simulink model "CRCL"  (R2020b)
settings: Solver=FixedStepDiscrete  StartTime=0.0  StopTime=inf  FixedStep=0.01  RelTol=1e-3  EnableMultiTasking=on
values from neighbouring files (symbols this model uses):
  calibrationDelayTime_s = 2.0    [CRCL_Dictionary.sldd]
  collisionAngleThreshold_deg = 40.0    [CRCL_Dictionary.sldd]
  collisionVarianceThreshold_g2 = 8.0    [CRCL_Dictionary.sldd]
  cpMaxAbortTime_s = 30.0    [CRCL_Dictionary.sldd]
  cpMaxTipOverAngle_deg = 35.0    [CRCL_Dictionary.sldd]
  cpMinEstDistance_m = 50.0    [CRCL_Dictionary.sldd]
  cpMinEstDistanceGnssBased_m = 200.0    [CRCL_Dictionary.sldd]
  cpMinRiddenTime_s = 15.0    [CRCL_Dictionary.sldd]
  cpMinSpeedRiding_kmh = 10.0    [CRCL_Dictionary.sldd]
  cpNumCrankRevolutionThreshold = 5.0    [CRCL_Dictionary.sldd]
  cpSpeedCond2PositiveSpeedChangeTime_s = 5.0    [CRCL_Dictionary.sldd]
  cpSpeedDerivativeThreshold_kmhs = 0.005    [CRCL_Dictionary.sldd]
  cpTimeOutSpeedCond2_s = 15.0    [CRCL_Dictionary.sldd]
  groundHitEnergyThresholdStanding_g2s2 = 0.02    [CRCL_Dictionary.sldd]
  groundHitTipOverAngleThreshold_deg = 40.0    [CRCL_Dictionary.sldd]
  longAccCompForEulerEstFlag = 0.0    [CRCL_Dictionary.sldd]
  minEnergyStrongHit_g2s2 = 0.1    [CRCL_Dictionary.sldd]
  noMotionAccVarianceThresholdSD_g2 = 0.001    [CRCL_Dictionary.sldd]
  ride1minSpeedSlow_kmh = 4.0    [CRCL_Dictionary.sldd]
  ride2minSpeed_kmh = 8.0    [CRCL_Dictionary.sldd]
  rroMaxSpeed_kmh = 5.0    [CRCL_Dictionary.sldd]
  rroMinGyrX_degs = 20.0    [CRCL_Dictionary.sldd]
  rroMonotonyThreshold_degs = -1.0    [CRCL_Dictionary.sldd]
  rroRollIntegrationAngleThreshold_degs = 20.0    [CRCL_Dictionary.sldd]
  rroUniContinuityThreshold_degs = 15.0    [CRCL_Dictionary.sldd]
  scaleFactorVarianceStrongHit = 2.0    [CRCL_Dictionary.sldd]
  sdoMaxAccVarFreeFall_g2 = 0.06    [CRCL_Dictionary.sldd]
  sdoMaxTipOverAngle_deg = 20.0    [CRCL_Dictionary.sldd]
  sdoMinAccVar_g2 = 8.0    [CRCL_Dictionary.sldd]
  sdoMinGyrXYNorm_degs = 720.0    [CRCL_Dictionary.sldd]
  sdoMinGyrXYNormFreeFall_degs = 100.0    [CRCL_Dictionary.sldd]
  sdoMinOrientationChange_deg = 120.0    [CRCL_Dictionary.sldd]
  sdoScaleFactorOrientationChange = 3.0    [CRCL_Dictionary.sldd]
  stepTime_s = 0.01    [CRCL_Dictionary.sldd]
  strongHitSafetyFactor = 2.5    [CRCL_Dictionary.sldd]
  tipOverAccZFiltTreshold_g = 0.7    [CRCL_Dictionary.sldd]
  tipOverAngleThreshold_deg = 50.0    [CRCL_Dictionary.sldd]
  tipOverMinAccZFiltNoseOver_g = 0.3    [CRCL_Dictionary.sldd]
  tipOverRollPitchRelationNoseOver = 1.5    [CRCL_Dictionary.sldd]
undefined symbols (not defined in the file or in its folder): magnitude
libraries: simulink x17
(part 1 of 8)
settings Model: DataDictionary=CRCL_Dictionary.sldd  EnableAccessToBaseWorkspace=off  DataTypeOverride=Off  DataTypeOverrideAppliesTo=Floating-point  MinMaxOverflowLogging=ForceOff  Creator=stj1si  LastModifiedBy=HNA3SI
settings DataIOCC: SaveFormat=Array  SaveOutput=off  SaveTime=off  ReturnWorkspaceOutputs=off
settings OptimizationCC: DefaultParameterBehavior=Inlined  DefaultUnderspecifiedDataType=single  InlineInvariantSignals=on  EnhancedBackFolding=on  CachingGlobalReferences=on  ExpressionDepthLimit=2147483647  NoFixptDivByZeroProtection=on  EfficientFloat2IntCast=on  LifeSpan=1  SimCompilerOptimization=on  EfficientTunableParamExpr=on
settings DebuggingCC: SolverPrmCheckMsg=warning  ParameterPrecisionLossMsg=none  AllowSymbolicDim=off  StateNameClashWarn=warning  SFUnexpectedBacktrackingDiag=warning  SFNoUnconditionalDefaultTransitionDiag=warning  SFExecutionAtInitializationDiag=none  UnderSpecifiedDimensionMsg=warning  ArithmeticOperatorsInVariantConditions=warning
settings HardwareCC: ProdBitPerPointer=32  ProdBitPerSizeT=32  ProdBitPerPtrDiffT=32  ProdLargestAtomicInteger=Long  ProdLargestAtomicFloat=Double  ProdEndianess=BigEndian  ProdWordSize=32  ProdHWDeviceType=Freescale->32-bit PowerPC
settings ModelReferenceCC: ModelReferenceNumInstancesAllowed=Single  PropagateSignalLabelsOutOfModel=off
settings SFSimCC: SimUseLocalCustomCode=off  MATLABDynamicMemAlloc=off  CustomCodeUndefinedFunction=UseInterfaceOnly
settings RTWCC: Description=Embedded Coder  SystemTargetFile=ert.tlc  GenCodeOnly=on  TemplateMakefile=ert_default_tmf  GenerateReport=on  RTWUseLocalCustomCode=off  IncludeHyperlinkInReport=on  LaunchReport=on  GenerateTraceInfo=on  GenerateTraceReport=on  GenerateTraceReportSl=on  GenerateTraceReportSf=on  GenerateTraceReportEml=on
settings CodeAppCC: IgnoreCustomStorageClasses=off  CustomSymbolStrType=$N$R$M  CustomSymbolStrBlkIO=SMON_rtb_$N$M  StateflowObjectComments=on  InternalIdentifier=Classic
settings ERTTargetCC: TargetLangStandard=C99 (ISO)  MultiwordLength=2048  GenerateSampleERTMain=on  IncludeMdlTerminateFcn=off  CombineSignalStateStructs=on  SuppressErrorStatus=on  SupportNonFinite=off  SupportComplex=off  CastingMode=Standards  InlinedParameterPlacement=NonHierarchical  ERTSrcFileBannerTemplate=ert_code_template_ebike.cgt  ERTCustomFileTemplate=example_file_process.tlc  ERTFilePackagingFormat=Compact  PreserveExternInFcnDecls=off  SuppressUnreachableDefaultCases=off  EnableSignedLeftShifts=off  EnableSignedRightShifts=off  IndentStyle=Allman  EnableUserReplacementTypes=on
settings ConfigComp: CovEnable=on  CovScope=ReferencedModels  CovIncludeTopModel=off  CovMetricSettings=dw  CovHTMLOptions=-sRT=1 -sVT=0 -aTS=1 -bRG=1 -bTC=1 -hTR=0 -nFC=0 -nFD=1 -scm=1 -bcm=1 -xEv=0 -xEM=0  CovSaveCumulativeToWorkspaceVar=on  CovSaveSingleToWorkspaceVar=on  CovModelRefEnable=all  CovSFcnEnable=off

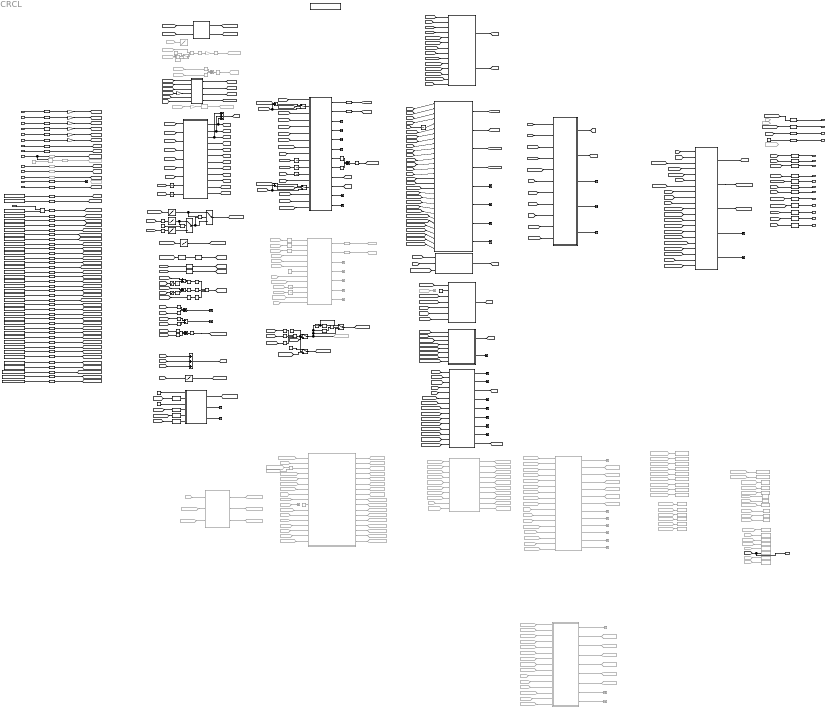
== system CRCL ==
  note: // hub setup (2==smarphoneHub, 1==bio bike cobi pro, 0==eBike cobi pro)
  note: remove speed jumps to 0km/h (FP Tobi 2021_03_30)
  note: set initially to 0.01s
  note: not used atm!
  note: RideDetection
  note: TipOverDetection
  note: HitAndStandDetection
  note: CrashFusion
  note: RiderlessRollOver
  note: SmartphoneDropOutDetection
  note: pass only current speed value, if hub Connection is available ( in eBike cobi use case)
  note: set initially to 2s
  note: set initially to 0 -> off
  note: set initially to 50°
  note: set initially to 0.3g
  note: set initially to 0.7g
  note: set initially to 1.5
  note: Cobi: set initially to 0.02
      | DU: set initially to 0.015 -> update!
  note: set initially to 40°
  note: set initially to 8g²
  note: Cobi: set initially to 2.5
      | DU: set initially to 3
  note: set initially to 2
  note: set initially to 0.1
  note: set initially to 40°
  note: set initially to 0.001 g²
  note: set initially to 4km/h
  note: set initially to 8km/h
  note: set initially to 20 °/s
  note: set initially to 15 °/s
  note: set initially to 5km/h
  note: set initially to -1°/s
  note: set initially to 20 °/s
  note: set initially to 20°
  note: set initially to 8g²
  note: set initially to 720°/s
  note: set initially to 120°
  note: set initially to 3
  note: set initially to 0.06g²
  note: set initially to 100°/s
  note: set initially to 5s
  note: set initially to 15s
  note: set initially to 15s
  note: set initially to 30s
  note: set initially to 5
  note: set initially to 200m
  note: set initially to 3 kmh
  note: set initially to 0.005 km/(h*s)
  note: set initially to 35°
  note: AVOID DIVISION BY ZERO!
  note: AVOID DIVISION BY ZERO!
  note: REMOVED DIVISION BY ZERO!
  note: Division by 0 possible!!!
  note: Division by 0 possible!!!
  note: AVOID DIVISION BY ZERO!
  note: not used atm!
  note: pass only current speed value, if hub Connection is avaiable ( in eBike cobi use case)
  note: set initially to 50m
  note: SystemConfig == 1 -> drive unit, SystemConfig == 2 -> all other
  acc_x [mg] : Inport  PortDimensions=1
  acc_y [mg] : Inport  Port=2  PortDimensions=1
  acc_z [mg] : Inport  Port=3  PortDimensions=1
  gyr_x [mdeg/s] : Inport  Port=4  PortDimensions=1
  gyr_y [mdeg/s] : Inport  Port=5  PortDimensions=1
  gyr_z [mdeg/s] : Inport  Port=6  PortDimensions=1
  DU_cadence [rpm] : Inport  Port=7  PortDimensions=1
  DU_Speed [kmh] : Inport  Port=8  PortDimensions=1
  SecondCalibDone : Inport  Port=9  PortDimensions=1
  SystemConfig [1/2] : Inport  Port=10  PortDimensions=1
  CobiHubConnection [0/1] : Inport  Port=11  PortDimensions=1
  cobiSetup [0/1/2] : Inport  Port=12  PortDimensions=1
  accDuX [mg] : Inport  Port=13  PortDimensions=1
  accDuZ [mg] : Inport  Port=14  PortDimensions=1
  speedCompFlag [0/1] : Inport  Port=15  PortDimensions=1
  1-D Lookup Table : Lookup_n-D  Commented=on  NumberOfTableDimensions=1  BreakpointsForDimension1=[1 2 3 4 5 6 7]  Table=[2 15 3 15 3 15 2]  ExtrapMethod=Clip  InternalRulePriority=Speed  RndMeth=Simplest  InputSameDT=on
  1-D Lookup Table1 : Lookup_n-D  NumberOfTableDimensions=1  BreakpointsForDimension1=[0 9000 10000 15000 30000 100000]  Table=[1 1 0.75 0.5 0.3 0.3]  InternalRulePriority=Speed  RndMeth=Simplest  InputSameDT=on
  1-D Lookup Table2 : Lookup_n-D  NumberOfTableDimensions=1  BreakpointsForDimension1=[0 20 35 45 50 90]  Table=[0.015 0.015 0.04 0.04 0.5 0.5]  InternalRulePriority=Speed  RndMeth=Simplest  InputSameDT=on
  1-D Lookup Table3 : Lookup_n-D  NumberOfTableDimensions=1  BreakpointsForDimension1=[0:100]  Table=-1./exp(0.09*[0:100]+3.5) + 0.045  InternalRulePriority=Speed  RndMeth=Simplest  InputSameDT=on
  1-D Lookup Table4 : Lookup_n-D  NumberOfTableDimensions=1  BreakpointsForDimension1=[0 20 45 60 180]  Table=[1 1 0.03 0.01 0.01]  InternalRulePriority=Speed  RndMeth=Simplest  InputSameDT=on
  1-D Lookup Table5 : Lookup_n-D  NumberOfTableDimensions=1  BreakpointsForDimension1=[0 15 25 90]  Table=[0.015 0.015 0.04 0.04]  InternalRulePriority=Speed  RndMeth=Simplest  InputSameDT=on
  Abs{,1..3,5} (5 alike) : Abs
  Abs4 : Abs  Commented=on
  Add : Sum  Inputs=+-
  Add1 : Sum  Inputs=+++
  Add10 : Sum  Inputs=-+
  Add2 : Sum  Commented=on
  Add{3..5,9} (4 alike) : Sum
  Add6 : Sum  Inputs=-+
  Add7 : Sum  Inputs=+++
  Add8 : Sum  Inputs=+-
  Atan : Trigonometry  Commented=on  Operator=atan
  BikeCrashFusionProduct : Stateflow chart  TreatAsAtomicUnit=on
  CP_crashPlausiblizer : Stateflow chart  TreatAsAtomicUnit=on
  Chart : Stateflow chart  TreatAsAtomicUnit=on
  Chart1 : Stateflow chart  TreatAsAtomicUnit=on
  Chart2 : Stateflow chart  Commented=on  TreatAsAtomicUnit=on
  Chart3 : Stateflow chart  Commented=on  TreatAsAtomicUnit=on
  Compare To Constant : simulink/Logic and Bit Operations/Compare To Constant  relop=>=  const=3  OutDataTypeStr=boolean
  Compare To Constant1 : simulink/Logic and Bit Operations/Compare To Constant  relop=>=  const=3  OutDataTypeStr=boolean
  Compare To Constant2 : simulink/Logic and Bit Operations/Compare To Constant  relop=>=  const=3  OutDataTypeStr=boolean
  Compare To Constant3 : simulink/Logic and Bit Operations/Compare To Constant  relop=<=  const=0.1  OutDataTypeStr=boolean
  Compare To Constant4 : simulink/Logic and Bit Operations/Compare To Constant  relop=>=  const=10  OutDataTypeStr=boolean
  Compare To Constant6 : simulink/Logic and Bit Operations/Compare To Constant  relop===  const=0  OutDataTypeStr=boolean
  Compare To Constant7 : simulink/Logic and Bit Operations/Compare To Constant  relop===  const=2  OutDataTypeStr=boolean
  Compare To Constant8 : simulink/Logic and Bit Operations/Compare To Constant  relop=~=  const=1  OutDataTypeStr=boolean
  Compare To Constant9 : simulink/Logic and Bit Operations/Compare To Constant  Commented=on  relop===  const=0  OutDataTypeStr=boolean
  Constant : Constant  Commented=on  Value=0.02  OutDataTypeStr=single
  Constant{1,7,9,11} (4 alike) : Constant  Value=0
  Constant10 : Constant  Value=tipOverAccZFiltTreshold_g
  Constant12 : Constant  Value=tipOverMinAccZFiltNoseOver_g
  Constant13 : Constant  Value=tipOverRollPitchRelationNoseOver
  Constant14 : Constant  Value=groundHitEnergyThresholdStanding_g2s2
  Constant15 : Constant  Value=minEnergyStrongHit_g2s2
  Constant16 : Constant  Value=collisionAngleThreshold_deg
  Constant17 : Constant  Value=noMotionAccVarianceThresholdSD_g2
  Constant18 : Constant  Value=ride1minSpeedSlow_kmh
  Constant19 : Constant  Value=groundHitTipOverAngleThreshold_deg
  Constant2 : Constant  Value=stepTime_s
  Constant20 : Constant  Value=collisionVarianceThreshold_g2
  Constant21 : Constant  Value=strongHitSafetyFactor
  Constant22 : Constant  Value=scaleFactorVarianceStrongHit
  Constant23 : Constant  Value=rroMonotonyThreshold_degs
  Constant24 : Constant  Value=rroRollIntegrationAngleThreshold_degs
  Constant25 : Constant  Value=sdoMaxTipOverAngle_deg
  Constant26 : Constant  Value=sdoMinAccVar_g2
  Constant27 : Constant  Value=sdoMinGyrXYNormFreeFall_degs
  Constant28 : Constant  Value=cpMaxAbortTime_s
  Constant29 : Constant  Value=cpMinSpeedRiding_kmh
  Constant3 : Constant  Value=calibrationDelayTime_s
  Constant30 : Constant  Value=cpNumCrankRevolutionThreshold
  Constant31 : Constant  Value=sdoMinGyrXYNorm_degs
  Constant32 : Constant  Value=ride2minSpeed_kmh
  Constant33 : Constant  Value=sdoMinOrientationChange_deg
  Constant34 : Constant  Value=sdoScaleFactorOrientationChange
  Constant35 : Constant  Value=sdoMaxAccVarFreeFall_g2
  Constant36 : Constant  Value=rroMinGyrX_degs
  Constant37 : Constant  Value=rroUniContinuityThreshold_degs
  Constant38 : Constant  Value=rroMaxSpeed_kmh
  Constant39 : Constant  Value=cpTimeOutSpeedCond2_s
  Constant4 : Constant  Commented=on
  Constant40 : Constant  Value=cpSpeedCond2PositiveSpeedChangeTime_s
  Constant41 : Constant  Value=cpSpeedDerivativeThreshold_kmhs
  Constant42 : Constant  Value=cpMaxTipOverAngle_deg
  Constant43 : Constant  Value=cpMinEstDistance_m
  Constant44 : Constant  Value=cpMinRiddenTime_s
  Constant45 : Constant  Commented=on  Value=0
  Constant46 : Constant  Value=10
  Constant47 : Constant  Value=0.1
  Constant48 : Constant  Commented=on  Value=0.001  OutDataTypeStr=single
  Constant49 : Constant  Value=0  OutDataTypeStr=single
  Constant5 : Constant  Value=longAccCompForEulerEstFlag
  Constant6 : Constant  Value=tipOverAngleThreshold_deg
  Constant8 : Constant  Value=cpMinEstDistanceGnssBased_m
  Data Type Conversion{,19,21,23..24,27..33} (12 alike) : DataTypeConversion  RndMeth=Zero
  Data Type Conversion{1..4,6..9,12..14,18,20,22,34..36,40,42..74,76..77} (53 alike) : DataTypeConversion  OutDataTypeStr=single
  Data Type Conversion10 : DataTypeConversion  RndMeth=Simplest
  Data Type Conversion11 : DataTypeConversion  OutDataTypeStr=int16
  Data Type Conversion15 : DataTypeConversion  OutDataTypeStr=Enum: CrashClass  RndMeth=Simplest
  Data Type Conversion16 : DataTypeConversion  RndMeth=Simplest
  Data Type Conversion17 : DataTypeConversion  RndMeth=Simplest
  Data Type Conversion25 : DataTypeConversion  Commented=on  OutDataTypeStr=single
  Data Type Conversion26 : DataTypeConversion  Commented=on  OutDataTypeStr=single
  Data Type Conversion{37..39,41} (4 alike) : DataTypeConversion  Commented=through  OutDataTypeStr=single
  Data Type Conversion5 : DataTypeConversion  Commented=on  OutDataTypeStr=single
  Data Type Conversion75 : DataTypeConversion  OutDataTypeStr=int16
  Discrete Derivative : simulink/Discrete/Discrete Derivative  gainval=1.0  ICPrevScaledInput=0.0  OutMin=[]  OutMax=[]  OutDataType=fixdt(1, 16)  OutScaling=2^-10  DoSatur=off
  Discrete Derivative1 : simulink/Discrete/Discrete Derivative  gainval=1.0  ICPrevScaledInput=0.0  OutMin=[]  OutMax=[]  OutDataType=fixdt(1, 16)  OutScaling=2^-10  DoSatur=off
  Discrete Derivative2 : simulink/Discrete/Discrete Derivative  gainval=1.0  ICPrevScaledInput=0.0  OutMin=[]  OutMax=[]  OutDataType=fixdt(1, 16)  OutScaling=2^-10  DoSatur=off
  Divide : Product  Commented=on  Inputs=*/
  Divide3 : Product  Commented=on  Inputs=*/
  Double-Click Button to set current folder : Subsystem
      settings: OpenFcn=cd(fileparts(get_param(gcs,'filename')));
      mask Display: disp('\bf\fontsize{16}Double-Click to set current folder      ','texmode','on')
  Environment Controller : simulink/Signal Routing/Environment Controller  Commented=on
      settings: SourceProductBaseCode=SL
  Environment Controller1 : simulink/Signal Routing/Environment Controller
      settings: SourceProductBaseCode=SL
  FilterButterworth : Subsystem
  From : From  Commented=on  GotoTag=CF_fire
  From101 : From  Commented=on  GotoTag=SecondCalibrationDone
  From102 : From  Commented=on  GotoTag=varSum
  From107 : From  Commented=on  GotoTag=speedDerivative
  From108 : From  Commented=on  GotoTag=accEnergyXY70ms
  From112 : From  Commented=on  GotoTag=accEnergyXY50ms
  From118 : From  Commented=on  GotoTag=accBfFiltX_g
  From119 : From  Commented=on  GotoTag=accBfFiltY_g
  From12 : From  Commented=on  GotoTag=CF_scenario
  From{120,188,192,197} (4 alike) : From  Commented=on  GotoTag=accBfFiltZ_g
  From139 : From  Commented=on  GotoTag=Du_Speed
  From140 : From  Commented=on  GotoTag=probRide1Latched
  From141 : From  Commented=on  GotoTag=probTipOverLatched
  From142 : From  Commented=on  GotoTag=probNoseOverLatched
  From143 : From  Commented=on  GotoTag=probRroLatched
  From{145,210,230,263} (4 alike) : From  Commented=on  GotoTag=tipOverAngle_deg
  From146 : From  Commented=on  GotoTag=SDO_fire
  From151 : From  Commented=on  GotoTag=reinitializeEulerEstimation
  From162 : From  Commented=on  GotoTag=hubConnection
  From163 : From  Commented=on  GotoTag=SystemConfig
  From164 : From  Commented=on  GotoTag=cobiHubSetup
  From{165,180,212,244} (4 alike) : From  Commented=on  GotoTag=SecondCalibrationDelayed
  From177 : From  Commented=on  GotoTag=tipOverAngleLatched
  From178 : From  Commented=on  GotoTag=accImpulseY
  From179 : From  Commented=on  GotoTag=rollDerivative
  From182 : From  Commented=on  GotoTag=groundHitScaleFactor
  From184 : From  Commented=on  GotoTag=eulerRoll_deg
  From185 : From  Commented=on  GotoTag=speedDerivative
  From186 : From  Commented=on  GotoTag=accBfFiltX_g
  From187 : From  Commented=on  GotoTag=accBfFiltY_g
  From191 : From  Commented=on  GotoTag=AccTipOverAngle_deg
  From193 : From  Commented=on  GotoTag=accBfFiltXY_g
  From194 : From  Commented=on  GotoTag=speed2sTransformRd
  From195 : From  Commented=on  GotoTag=TO_fire
  From196 : From  Commented=on  GotoTag=AccTipOverAngle_deg
  From198 : From  Commented=on  GotoTag=eulerPitch_deg
  From199 : From  Commented=on  GotoTag=eulerRoll_deg
  From200 : From  Commented=on  GotoTag=speedDerivativeTransformRd
  From201 : From  Commented=on  GotoTag=accEnergyXY70ms
  From202 : From  Commented=on  GotoTag=speedTransformCollision
  From203 : From  Commented=on  GotoTag=tipOverAngleTransformCollision
  From204 : From  Commented=on  GotoTag=accEnergyXY50ms
  From205 : From  Commented=on  GotoTag=tipOverAngleFusedTransformTO
  From206 : From  Commented=on  GotoTag=tipOverAngleAccTransformTO
  From207 : From  Commented=on  GotoTag=pitchAngleTransformTO2
  From208 : From  Commented=on  GotoTag=pitchRollRelationTransformTO2
  From209 : From  Commented=on  GotoTag=accBfZTransformTO2
  From211 : From  Commented=on  GotoTag=HD_CollisionFire
  From213 : From  Commented=on  GotoTag=probColl
  From214 : From  Commented=on  GotoTag=probStrongColl
  From215 : From  Commented=on  GotoTag=probSoftColl
  From216 : From  Commented=on  GotoTag=probGroundHit
  From217 : From  Commented=on  GotoTag=probRide1
  From218 : From  Commented=on  GotoTag=probRide2
  From219 : From  Commented=on  GotoTag=probTipOver
  From220 : From  Commented=on  GotoTag=probNoseOver
  From221 : From  Commented=on  GotoTag=probRide2Latched
  From222 : From  Commented=on  GotoTag=probGroundHitLatched
  From223 : From  Commented=on  GotoTag=probSoftCollLatched
  From224 : From  Commented=on  GotoTag=probCollLatched
  From225 : From  Commented=on  GotoTag=probStrongCollLatched
  From226 : From  Commented=on  GotoTag=probRide1Latched
  From227 : From  Commented=on  GotoTag=probTipOverLatched
  From228 : From  Commented=on  GotoTag=probNoseOverLatched
  From229 : From  Commented=on  GotoTag=probRroLatched
  From231 : From  Commented=on  GotoTag=finalProbCrashClass
  From232 : From  Commented=on  GotoTag=SDO_fire
  From233 : From  Commented=on  GotoTag=hubConnection
  From234 : From  Commented=on  GotoTag=SystemConfig
  From235 : From  Commented=on  GotoTag=crashProbability
  From236 : From  Commented=on  GotoTag=probCrashClass
  From237 : From  Commented=on  GotoTag=curMostProbCrashClass
  From238 : From  Commented=on  GotoTag=AccTipOverAngle_deg
  From239 : From  Commented=on  GotoTag=RRO_fire
  From241 : From  Commented=on  GotoTag=cobiHubSetup
  From242 : From  Commented=on  GotoTag=generalCrashClass
  From243 : From  Commented=on  GotoTag=probGeneralCrashClass
  From249 : From  Commented=on  GotoTag=varSum
  From25 : From  Commented=on  GotoTag=probRide2Latched
  From250 : From  Commented=on  GotoTag=accEnergyXY70ms
  From251 : From  Commented=on  GotoTag=accVarianceLatched
  From252 : From  Commented=on  GotoTag=accXYEnergy70msLatched
  From253 : From  Commented=on  GotoTag=accBfFiltX_g
  From254 : From  Commented=on  GotoTag=accBfFiltY_g
  From255 : From  Commented=on  GotoTag=duAccZ_mg
  From259 : From  Commented=on  GotoTag=HD_GroundHitFire
  From26 : From  Commented=on  GotoTag=probGroundHitLatched
  From260 : From  Commented=on  GotoTag=RD_fire
  From262 : From  Commented=on  GotoTag=SDO_fire
  From265 : From  Commented=on  GotoTag=SD_fire
  From273 : From  Commented=on  GotoTag=probTipOverTimer
  From276 : From  Commented=on  GotoTag=SDO_bikeStillUpright
  From277 : From  Commented=on  GotoTag=cobiHubSetup
  From278 : From  Commented=on  GotoTag=SystemConfig
  From279 : From  Commented=on  GotoTag=duAccZFiltToG
  From280 : From  Commented=on  GotoTag=CF_confidenceLevel
  From33 : From  Commented=on  GotoTag=CP_plausibleCrashFire
  From49 : From  Commented=on  GotoTag=probSoftCollLatched
  From50 : From  Commented=on  GotoTag=probCollLatched
  From51 : From  Commented=on  GotoTag=probStrongCollLatched
  From52 : From  Commented=on  GotoTag=BMI_GYR_BF_X
  From53 : From  Commented=on  GotoTag=BMI_GYR_BF_Y
  From54 : From  Commented=on  GotoTag=BMI_GYR_BF_Z
  From57 : From  Commented=on  GotoTag=SD_fire
  From69 : From  Commented=on  GotoTag=CP_scenario
  From70 : From  Commented=on  GotoTag=HD_GroundHitFire
  From72 : From  Commented=on  GotoTag=eulerPitch_deg
  From73 : From  Commented=on  GotoTag=dataSource
  From9 : From  Commented=on  GotoTag=HD_CollisionFire
  Gain{,1..2,4..6,9} (7 alike) : Gain  Gain=1/1000
  Gain12 : Gain  Commented=on  Gain=180/pi
  Gain8 : Gain  Commented=on  Gain=1/1000
  Goto1 : Goto  Commented=on  GotoTag=SecondCalibrationDone
  Goto102 : Goto  Commented=on  GotoTag=probGeneralCrashClass
  Goto103 : Goto  Commented=on  GotoTag=generalCrashClass
  Goto110 : Goto  Commented=on  GotoTag=accVarianceLatched
  Goto111 : Goto  Commented=on  GotoTag=accXYEnergy70msLatched
  Goto112 : Goto  Commented=on  GotoTag=duAccX_mg
  Goto114 : Goto  Commented=on  GotoTag=duAccZFiltToG
  Goto154 : Goto  Commented=on  GotoTag=validatedSpeed_kmh
  Goto3 : Goto  Commented=on  GotoTag=probGeneralCrashClass
  Goto33 : Goto  Commented=on  GotoTag=eulerPitch_deg
  Goto34 : Goto  Commented=on  GotoTag=eulerRoll_deg
  Goto35 : Goto  Commented=on  GotoTag=tipOverAngleLatched
  Goto4 : Goto  Commented=on  GotoTag=generalCrashClass
  Goto50 : Goto  Commented=on  GotoTag=finalProbCrashClass
  Goto51 : Goto  Commented=on  GotoTag=crashProbability
  Goto52 : Goto  Commented=on  GotoTag=probCrashClass
  Goto59 : Goto  Commented=on  GotoTag=curMostProbCrashClass
  Goto63 : Goto  Commented=on  GotoTag=accBfFiltXY_g
  Goto66 : Goto  Commented=on  GotoTag=AccTipOverAngle_deg
  Goto67 : Goto  Commented=on  GotoTag=tipOverAngleFusedTransformTO
  Goto68 : Goto  Commented=on  GotoTag=probTipOverTimer
  Goto70 : Goto  Commented=on  GotoTag=tipOverAngleTransformCollision
  Goto71 : Goto  Commented=on  GotoTag=speedTransformCollision
  Goto72 : Goto  Commented=on  GotoTag=speed2sTransformRd
  Goto73 : Goto  Commented=on  GotoTag=speedDerivativeTransformRd
  Goto74 : Goto  Commented=on  GotoTag=tipOverAngleAccTransformTO
  Goto75 : Goto  Commented=on  GotoTag=pitchAngleTransformTO2
  Goto76 : Goto  Commented=on  GotoTag=pitchRollRelationTransformTO2
  Goto77 : Goto  Commented=on  GotoTag=accBfZTransformTO2
  Goto78 : Goto  Commented=on  GotoTag=probColl
  Goto79 : Goto  Commented=on  GotoTag=probStrongColl
  Goto80 : Goto  Commented=on  GotoTag=probSoftColl
  Goto81 : Goto  Commented=on  GotoTag=probGroundHit
  Goto82 : Goto  Commented=on  GotoTag=probRide1
  Goto83 : Goto  Commented=on  GotoTag=probRide2
  Goto84 : Goto  Commented=on  GotoTag=probTipOver
  Goto85 : Goto  Commented=on  GotoTag=probNoseOver
  Goto86 : Goto  Commented=on  GotoTag=probCollLatched
  Goto87 : Goto  Commented=on  GotoTag=probStrongCollLatched
  Goto88 : Goto  Commented=on  GotoTag=probSoftCollLatched
  Goto89 : Goto  Commented=on  GotoTag=probGroundHitLatched
  Goto90 : Goto  Commented=on  GotoTag=probRide1Latched
  Goto91 : Goto  Commented=on  GotoTag=probRide2Latched
  Goto92 : Goto  Commented=on  GotoTag=probTipOverLatched
  Goto93 : Goto  Commented=on  GotoTag=probNoseOverLatched
  Goto94 : Goto  Commented=on  GotoTag=finalProbCrashClass
  Goto96 : Goto  Commented=on  GotoTag=crashProbability
  Goto97 : Goto  Commented=on  GotoTag=probCrashClass
  Goto98 : Goto  Commented=on  GotoTag=curMostProbCrashClass
  Goto99 : Goto  Commented=on  GotoTag=probRroLatched
  HitDetection : Stateflow chart  TreatAsAtomicUnit=on
  Logical Operator : Logic  AllPortsSameDT=off  OutDataTypeStr=boolean
  Logical Operator1 : Logic  Operator=OR  Inputs=3  AllPortsSameDT=off  OutDataTypeStr=boolean
  Logical Operator2 : Logic  Inputs=3  AllPortsSameDT=off  OutDataTypeStr=boolean
  MATLAB Function : MATLAB Function  TreatAsAtomicUnit=on
  MATLAB Function1 : MATLAB Function  Commented=on  TreatAsAtomicUnit=on
  MATLAB Function2 : MATLAB Function  TreatAsAtomicUnit=on
  MATLAB Function5 : MATLAB Function  Commented=on  TreatAsAtomicUnit=on
  MATLAB Function6 : MATLAB Function  Commented=on  TreatAsAtomicUnit=on
  Madgwick IMU MATLAB Function1 : MATLAB Function  Commented=on  TreatAsAtomicUnit=on
  Math Function : Math  Commented=on  Operator=magnitude^2  SignedPower=on  SaturateOnIntegerOverflow=on
  Math Function1 : Math  Commented=on  Operator=magnitude^2  SignedPower=on  SaturateOnIntegerOverflow=on
  Math Function{2..7} (6 alike) : Math  Operator=magnitude^2  SignedPower=on  SaturateOnIntegerOverflow=on
  Relational Operator : RelationalOperator  Operator=>  OutDataTypeStr=boolean  RndMeth=Simplest
  Relational Operator1 : RelationalOperator  Operator=>  OutDataTypeStr=boolean  RndMeth=Simplest
  RideDetection_RD : Stateflow chart  TreatAsAtomicUnit=on
  Saturation : Saturate  UpperLimit=3  LowerLimit=-3
  Saturation1 : Saturate  UpperLimit=3  LowerLimit=-3
  SmartphoneDropOut_SDO : Stateflow chart  TreatAsAtomicUnit=on
  Sqrt : Sqrt  Commented=on  SaturateOnIntegerOverflow=on
  Sqrt1 : Sqrt  SaturateOnIntegerOverflow=on
  Sqrt2 : Sqrt  SaturateOnIntegerOverflow=on
  Square : Math  Operator=square  SignedPower=on  SaturateOnIntegerOverflow=on
  Square1 : Math  Operator=square  SignedPower=on  SaturateOnIntegerOverflow=on
  StandDetection_SD : Stateflow chart  TreatAsAtomicUnit=on
  Switch{,1..6} (7 alike) : Switch  Criteria=u2 > Threshold
  Switch7 : Switch  Commented=on  Criteria=u2 > Threshold
  Terminator{,1..19,35,38..44} (28 alike) : Terminator
  Terminator{20..34,36..37} (17 alike) : Terminator  Commented=on
  TipOver : Stateflow chart  TreatAsAtomicUnit=on
  To Workspace1 : ToWorkspace  Commented=on  VariableName=accLpfBfY_g  SampleTime=-1
  To Workspace10 : ToWorkspace  Commented=on  VariableName=tipOverAngleTransformCollision  SampleTime=-1
  To Workspace11 : ToWorkspace  Commented=on  VariableName=accEnergyXY70ms  SampleTime=-1
  To Workspace12 : ToWorkspace  Commented=on  VariableName=accEnergyXY50ms  SampleTime=-1
  To Workspace13 : ToWorkspace  Commented=on  VariableName=tipOverAngleFusedTransformTO  SampleTime=-1
  To Workspace14 : ToWorkspace  Commented=on  VariableName=tipOverAngleAccTransformTO  SampleTime=-1
  To Workspace15 : ToWorkspace  Commented=on  VariableName=pitchAngleTransformTO2  SampleTime=-1
  To Workspace16 : ToWorkspace  Commented=on  VariableName=pitchRollRelationTransformTO2  SampleTime=-1
  To Workspace17 : ToWorkspace  Commented=on  VariableName=accBfZTransformTO2  SampleTime=-1
  To Workspace18 : ToWorkspace  Commented=on  VariableName=tipOverAngleFused  SampleTime=-1
  To Workspace19 : ToWorkspace  Commented=on  VariableName=crashScenario  SampleTime=-1
  To Workspace2 : ToWorkspace  Commented=on  VariableName=accLpfBfZ_g  SampleTime=-1
  To Workspace20 : ToWorkspace  Commented=on  VariableName=calibrationState  SampleTime=-1
  To Workspace21 : ToWorkspace  Commented=on  VariableName=finalProbCrashClass  SampleTime=-1
  To Workspace22 : ToWorkspace  Commented=on  VariableName=crashProbability  SampleTime=-1
  To Workspace23 : ToWorkspace  Commented=on  VariableName=probCrashClass  SampleTime=-1
  To Workspace24 : ToWorkspace  Commented=on  VariableName=curMostProbCrashClass  SampleTime=-1
  To Workspace25 : ToWorkspace  Commented=on  VariableName=generalCrashClass  SampleTime=-1
  To Workspace26 : ToWorkspace  Commented=on  VariableName=probGeneralCrashClass  SampleTime=-1
  To Workspace27 : ToWorkspace  Commented=on  VariableName=crashFire  SampleTime=-1
  To Workspace28 : ToWorkspace  Commented=on  VariableName=collisionFire  SampleTime=-1
  To Workspace29 : ToWorkspace  Commented=on  VariableName=rollAngle_deg  SampleTime=-1
  To Workspace30 : ToWorkspace  Commented=on  VariableName=pitchAngle_deg  SampleTime=-1
  To Workspace31 : ToWorkspace  Commented=on  VariableName=groundHitFire  SampleTime=-1
  To Workspace32 : ToWorkspace  Commented=on  VariableName=rdFire  SampleTime=-1
  To Workspace33 : ToWorkspace  Commented=on  VariableName=rroFire  SampleTime=-1
  To Workspace34 : ToWorkspace  Commented=on  VariableName=sdoFire  SampleTime=-1
  To Workspace35 : ToWorkspace  Commented=on  VariableName=sdFire  SampleTime=-1
  To Workspace4 : ToWorkspace  Commented=on  VariableName=accLpfBfX_g  SampleTime=-1
  To Workspace5 : ToWorkspace  Commented=on  VariableName=accTipOverAngle_deg  SampleTime=-1
  To Workspace6 : ToWorkspace  Commented=on  VariableName=toFire  SampleTime=-1
  To Workspace7 : ToWorkspace  Commented=on  VariableName=speed2sTransformRD  SampleTime=-1
  To Workspace8 : ToWorkspace  Commented=on  VariableName=speedDerivativeTransformRd  SampleTime=-1
  To Workspace9 : ToWorkspace  Commented=on  VariableName=speedTransformCollision  SampleTime=-1
  Transfer Fcn First Order : simulink/Discrete/Transfer Fcn First Order  PoleZ=0.995  ICPrevOutput=0.0  DoSatur=off
  Transfer Fcn First Order1 : simulink/Discrete/Transfer Fcn First Order  Commented=on  PoleZ=0.99  ICPrevOutput=1.0  DoSatur=off
  Unit Delay{,3..10} (9 alike) : UnitDelay  SampleTime=-1  HasFrameUpgradeWarning=on
  Unit Delay{1..2,13..15} (5 alike) : UnitDelay  Commented=on  SampleTime=-1  HasFrameUpgradeWarning=on
  risingEdgeTrigger_RET : Stateflow chart  TreatAsAtomicUnit=on
  CRCL_fire [0/1] : Outport  VectorParamsAs1DForOutWhenUnconnected=off
  CRCL_sceanrio [0-9] : Outport  Port=2  VectorParamsAs1DForOutWhenUnconnected=off
  CRCL_abort [0/1] : Outport  Port=3  VectorParamsAs1DForOutWhenUnconnected=off
  CRCL_confidenceLevel [0-1] : Outport  Port=4  VectorParamsAs1DForOutWhenUnconnected=off
  TO_fire [0/1] : Outport  Port=5  VectorParamsAs1DForOutWhenUnconnected=off
  TO_curAngle [°] : Outport  Port=6  VectorParamsAs1DForOutWhenUnconnected=off
  HD_groundHitFire  [0/1] : Outport  Port=7  VectorParamsAs1DForOutWhenUnconnected=off
  HD_collisionHitFire  [0/1] : Outport  Port=8  VectorParamsAs1DForOutWhenUnconnected=off
  HD_collisionHitCurVarSum  [] : Outport  Port=9  VectorParamsAs1DForOutWhenUnconnected=off
  SD_fire  [0/1] : Outport  Port=10  VectorParamsAs1DForOutWhenUnconnected=off
  RD_fire  [0/1] : Outport  Port=11  VectorParamsAs1DForOutWhenUnconnected=off
  HD_hitDirection  [1-4] : Outport  Port=12  VectorParamsAs1DForOutWhenUnconnected=off
  SecondCalibrationDelayed [0/1] : Outport  Port=13  VectorParamsAs1DForOutWhenUnconnected=off
  eulerPitch [°] : Outport  Port=14  VectorParamsAs1DForOutWhenUnconnected=off
  eulerRoll [°] : Outport  Port=15  VectorParamsAs1DForOutWhenUnconnected=off
  SmartphoneDropOutFire [0/1/2] : Outport  Port=16  VectorParamsAs1DForOutWhenUnconnected=off
  RRO_fire [0/1] : Outport  Port=17  VectorParamsAs1DForOutWhenUnconnected=off
  wires:
  acc_y [mg]/1 -> Data Type Conversion3/1  "ROID_accBfYMg"
  acc_x [mg]/1 -> Data Type Conversion2/1  "ROID_accBfXMg"
  Data Type Conversion2/1 -> Gain/1  "accBfX_mg"
  Data Type Conversion3/1 -> Gain1/1  "accBfY_mg"
  Data Type Conversion1/1 -> Gain2/1  "accBfZ_mg"
  acc_z [mg]/1 -> Data Type Conversion1/1  "ROID_accBfZMg"
  gyr_x [mdeg/s]/1 -> Data Type Conversion8/1  "ROID_gyrBfXMdegs"
  gyr_y [mdeg/s]/1 -> Data Type Conversion9/1  "ROID_gyrBfYMdegs"
  Data Type Conversion9/1 -> Gain5/1  "gyrBfY_mdegs"
  Data Type Conversion7/1 -> Gain6/1  "gyrBfZ_mdegs"
  Data Type Conversion8/1 -> Gain4/1  "gyrBfX_mdegs"
  gyr_z [mdeg/s]/1 -> Data Type Conversion7/1  "ROID_gyrBfZMdegs"
  Data Type Conversion10/1 -> CRCL_fire [0/1]/1  "CRCL_fire"
  Data Type Conversion15/1 -> CRCL_sceanrio [0-9]/1  "CRCL_scenario"
  Data Type Conversion16/1 -> CRCL_abort [0/1]/1  "CRCL_abort"
  Data Type Conversion17/1 -> CRCL_confidenceLevel [0-1]/1  "CRCL_confidenceLevel"
  Add1/1 -> [varSum]  "accVarSum"
  Unit Delay4/1 -> MATLAB Function2/8(roll_deg)
  MATLAB Function2/3(varAccZ) -> Add1/1, [accVarZ]  "varAccZ"
  Abs/1 -> Compare To Constant/1
  HitDetection/4(HD_hitDirection) -> [HD_HitDirection]  "HD_HitDirection"
  Compare To Constant2/1 -> Logical Operator1/3
  Compare To Constant1/1 -> Logical Operator1/2
  [SecondCalibrationDelayed] -> BikeCrashFusionProduct/5(HD_secondCalibrationDone)
  BikeCrashFusionProduct/1(CF_fire) -> [CF_fire]  "CF_fire"
  Compare To Constant/1 -> Logical Operator1/1
  Abs2/1 -> Compare To Constant2/1
  [BMI_GYR_BF_X] -> Add8/1
  [BMI_GYR_BF_Z] -> Abs2/1
  Unit Delay14/1 -> Madgwick IMU MATLAB Function1/2(AccelerometerY)
  MATLAB Function2/12(impulseShortTermY) -> [accImpulseSTY]  "impulseSTY"
  HitDetection/3(HD_CollisionCurVarSum) -> [HD_CollisionCurVarSum]  "HD_CollisionCurVarSum"
  HitDetection/5(HD_collisionFrontalRearLat) -> Terminator40/1  "HD_collisionFrontalRearLat"
  [accVarZ] -> HitDetection/3(HD_curVarZ)
  MATLAB Function2/11(impulseShortTermX) -> [accImpulseSTX]  "impulseSTX"
  [validatedSpeed_kmh] -> HitDetection/18(HD_curSpeed_kmh)
  From9/1 -> Unit Delay2/1
  Abs1/1 -> Compare To Constant1/1
  Madgwick IMU MATLAB Function1/2(eulerRoll) -> Data Type Conversion25/1  "rollMadgwick_deg"
  MATLAB Function2/7(impulseX) -> [accImpulseX]  "impulseX"
  From53/1 -> Madgwick IMU MATLAB Function1/5(gyrBfY)
  HitDetection/2(HD_collisionHitFire) -> [HD_CollisionFire]  "HD_CollisionHitFire"
  [eulerPitch_deg] -> Unit Delay5/1
  [accImpulseSTX] -> HitDetection/16(HD_curAccImpulseSTX)
  [accImpulseSTY] -> HitDetection/17(HD_curAccImpulseSTY)
  [BMI_GYR_BF_Y] -> Add/1
  HitDetection/6(HD_softCollisionHitFireTmp) -> Terminator6/1  "softCollisionTmp"
  From118/1 -> Unit Delay13/1
  Unit Delay13/1 -> Madgwick IMU MATLAB Function1/1(AccelerometerX)
  Unit Delay15/1 -> Madgwick IMU MATLAB Function1/3(AccelerometerZ)
  [accImpulseZ] -> HitDetection/11(HD_curAccImpulseZ)
  TipOver/2(TO_curAngle) -> [TO_curAngle]  "TO_curAngle"
  [eulerRoll_deg] -> Unit Delay4/1
  From101/1 -> Madgwick IMU MATLAB Function1/12(SecondCalibrationDone)
  Discrete Derivative1/1 -> [pitchDerivative]  "PitchDerivative"
  MATLAB Function2/10(extremaAccValY) -> [maxAccValY]  "maxAccY"
  Constant/1 -> Madgwick IMU MATLAB Function1/7(Beta)
  [eulerPitch_deg] -> Discrete Derivative1/1
  [pitchDerivative] -> HitDetection/13(HD_curPitchDeriv)
  From119/1 -> Unit Delay14/1
  MATLAB Function2/9(impulseZ) -> [accImpulseZ]  "impulseZ"
  [rollDerivative] -> HitDetection/12(HD_curRollDeriv)
  [eulerRoll_deg] -> Discrete Derivative/1
  StandDetection_SD/1(SD_StandFire) -> [SD_fire]  "SD_StandFire"
  Discrete Derivative/1 -> [rollDerivative]  "RollDerivative"
  [accVarX] -> HitDetection/1(HD_curVarX)
  [maxAccValY] -> HitDetection/14(HD_curAccYMax)
  [accBfY_g] -> HitDetection/7(HD_curAccBfY)
  From70/1 -> Unit Delay1/1
  BikeCrashFusionProduct/2(CF_scenario) -> [CF_scenario]  "CF_scenario"
  [StepTime] -> MATLAB Function2/7(stepTime_s)
  MATLAB Function2/8(impulseY) -> [accImpulseY]  "impulseY"
  [accVarY] -> HitDetection/2(HD_curVarY)
  From120/1 -> Unit Delay15/1
  Unit Delay5/1 -> MATLAB Function2/9(pitch_deg)
  MATLAB Function2/1(varAccX) -> Add1/3, [accVarX]  "varAccX"
  Madgwick IMU MATLAB Function1/1(eulerPitch) -> Data Type Conversion26/1  "pitchMadgwick_deg"
  MATLAB Function2/2(varAccY) -> Add1/2, [accVarY]  "varAccY"
  TipOver/1(TO_fire) -> [TO_fire]  "TO_fire"
  [accImpulseX] -> HitDetection/9(HD_curAccImpulseX)
  [accImpulseY] -> HitDetection/10(HD_curAccImpulseY)
  From52/1 -> Madgwick IMU MATLAB Function1/4(gyrBfX)
  From54/1 -> Madgwick IMU MATLAB Function1/6(gyrBfZ)
  [StepTime] -> TipOver/2(timestep)
  [RD_fire] -> BikeCrashFusionProduct/2(RD_fire)
  RideDetection_RD/1(RD_fire) -> [RD_fire]  "RD_fire"
  [accBfX_g] -> HitDetection/6(HD_curAccBfX)
  [HD_GroundHitFire] -> BikeCrashFusionProduct/4(HD_GroundHitFire)
  [HD_CollisionFire] -> BikeCrashFusionProduct/3(HD_CollisionHitFire)
  [TO_fire] -> BikeCrashFusionProduct/1(TO_fire)
  [accBfY_g] -> HitDetection/8(HD_curAccBfZ)
  HitDetection/1(HD_groundHitFire) -> [HD_GroundHitFire]  "HD_GroundHitFire"
  [TO_fire] -> HitDetection/4(HD_curTipOverFire)
  Data Type Conversion5/1 -> Goto1/1
  Constant4/1 -> Environment Controller/2
  Gain/1 -> [accBfX_g]  "accBfX_g"
  Gain1/1 -> [accBfY_g]  "accBfY_g"
  Gain2/1 -> [accBfZ_g]  "accBfZ_g"
  Constant2/1 -> Data Type Conversion4/1  "stepTime_s"
  DU_Speed [kmh]/1 -> Data Type Conversion13/1  "SPECO_getPresentSpeed"
  Data Type Conversion20/1 -> [Du_Cadence]  "DriverCadence_rpm"
  DU_cadence [rpm]/1 -> Data Type Conversion20/1  "CADE_getDriverCadence"
  Data Type Conversion13/1 -> [Du_Speed]  "DuSpeed_kmh"
  Gain4/1 -> [BMI_GYR_BF_X]  "gyrBfX_degs"
  Gain5/1 -> [BMI_GYR_BF_Y]  "gyrBfY_degs"
  Gain6/1 -> [BMI_GYR_BF_Z]  "gyrBfZ_degs"
  Logical Operator1/1 -> [gyrMotionFlag]  "gyrMotion"
  [gyrMotionFlag] -> StandDetection_SD/1(SD_curGyrMotion)
  [eulerPitch_deg] -> TipOver/4(TO_curPitch_deg)
  [eulerRoll_deg] -> TipOver/3(TO_curRoll_deg)
  [varSum] -> StandDetection_SD/2(SD_curVarSum)
  Constant1/1 -> Data Type Conversion17/1
  [CP_abort] -> Data Type Conversion16/1
  Data Type Conversion26/1 -> Goto33/1
  Data Type Conversion25/1 -> Goto34/1
  From57/1 -> Madgwick IMU MATLAB Function1/8(SD_fire)
  Unit Delay1/1 -> Madgwick IMU MATLAB Function1/10(HD_GroundHit)
  Unit Delay2/1 -> Madgwick IMU MATLAB Function1/11(HD_CollisionHit)
  From102/1 -> Madgwick IMU MATLAB Function1/13(curVarSum)
  Environment Controller/1 -> Data Type Conversion5/1
  SecondCalibDone/1 -> Data Type Conversion37/1, Environment Controller/1  "ROID_calibrationStatus"
  [TO_fire] -> Data Type Conversion/1
  [TO_curAngle] -> Data Type Conversion19/1
  [HD_GroundHitFire] -> Data Type Conversion21/1
  [HD_CollisionFire] -> Data Type Conversion23/1
  Data Type Conversion/1 -> TO_fire [0/1]/1
  Data Type Conversion19/1 -> TO_curAngle [°]/1
  Data Type Conversion21/1 -> HD_groundHitFire  [0/1]/1
  Data Type Conversion23/1 -> HD_collisionHitFire  [0/1]/1
  [HD_CollisionCurVarSum] -> Data Type Conversion24/1
  Data Type Conversion24/1 -> HD_collisionHitCurVarSum  []/1
  [HD_HitDirection] -> Data Type Conversion29/1
  [RD_fire] -> Data Type Conversion28/1
  [SD_fire] -> Data Type Conversion27/1
  Data Type Conversion27/1 -> SD_fire  [0/1]/1
  Data Type Conversion28/1 -> RD_fire  [0/1]/1
  Data Type Conversion29/1 -> HD_hitDirection  [1-4]/1
  [SecondCalibrationDelayed] -> Data Type Conversion30/1
  Data Type Conversion30/1 -> SecondCalibrationDelayed [0/1]/1
  [eulerPitch_deg] -> Data Type Conversion31/1
  [eulerRoll_deg] -> Data Type Conversion32/1
  Data Type Conversion31/1 -> eulerPitch [°]/1
  Data Type Conversion32/1 -> eulerRoll [°]/1
  [BMI_GYR_BF_X] -> Chart/1(RRO_curGyrX)
  Chart/1(RRO_fire) -> [RRO_fire]  "RRO_fire"
  [StepTime] -> Chart/2(steptime_s)
  [RRO_fire] -> BikeCrashFusionProduct/6(RRO_fire)
  [SecondCalibrationDone] -> HitDetection/19(HD_secCalibDone)
  [validatedSpeed_kmh] -> Chart/3(RRO_curSpeed_kmh)
  [validatedSpeed_kmh] -> 1-D Lookup Table3/1
  [CollisionEnergyThreshold] -> HitDetection/20(HD_CollisionEnergyThreshold)
  1-D Lookup Table3/1 -> Relational Operator/1, Switch/1  "CollisionEnergyThresholdSpeed"
  HitDetection/7(HD_varThres) -> Terminator7/1  "accVarThresStrongHit"
  Data Type Conversion37/1 -> [SecondCalibrationDone]  "calibrationStatus"
  Madgwick IMU MATLAB Function1/4(BetaIntern) -> Terminator21/1  "BetaInternCrashModul"
  [SecondCalibrationDelayed] -> TipOver/6(TO_CalibrationStatus)
  Data Type Conversion38/1 -> [SystemConfig]  "SystemConfig"
  SystemConfig [1/2]/1 -> Data Type Conversion38/1  "CRCL_systemConfig"
  [SystemConfig] -> BikeCrashFusionProduct/7(CF_systemConfig)
  CobiHubConnection [0/1]/1 -> Data Type Conversion39/1  "CRCL_CobiHubConnection"
  Data Type Conversion39/1 -> [hubConnection]  "cobiHubConnection"
  [eulerRoll_deg] -> Abs3/1
  Switch/1 -> [CollisionEnergyThreshold]  "CollisionEnergyThreshold"
  Relational Operator/1 -> Switch/2
  [hubConnection] -> BikeCrashFusionProduct/8(CF_hubConnection)
  BikeCrashFusionProduct/3(RD_fireIntern) -> Terminator17/1  "RD_fireIntern"
  BikeCrashFusionProduct/4(CF_possibleTo) -> Terminator18/1  "possibleTO"
  [StepTime] -> SmartphoneDropOut_SDO/1(SDO_timestep)
  [BMI_GYR_BF_Y] -> SmartphoneDropOut_SDO/3(SDO_curGyroBfY)
  [BMI_GYR_BF_X] -> SmartphoneDropOut_SDO/2(SDO_curGyroBfX)
  SmartphoneDropOut_SDO/3(SDO_fire) -> [SDO_fire]  "SDO_fire"
  SmartphoneDropOut_SDO/1(SDO_deltaRoll_deg) -> Terminator10/1  "deltaRoll_deg"
  SmartphoneDropOut_SDO/2(SDO_deltaPitch_deg) -> Terminator11/1  "deltaPitch_deg"
  SmartphoneDropOut_SDO/4(SDO_gyrXYnorm) -> Terminator12/1  "gyrXYnorm"
  [validatedSpeed_kmh] -> Transfer Fcn First Order/1
  Transfer Fcn First Order/1 -> Discrete Derivative2/1  "speedFilt_kmh"
  Discrete Derivative2/1 -> [speedDerivative]  "CRCL_speedDerivative"
  [SDO_fire] -> Data Type Conversion33/1
  Data Type Conversion33/1 -> SmartphoneDropOutFire [0/1/2]/1  "CRCL_SdoFire"
  [accBfZ_g] -> FilterButterworth/3(Z)
  FilterButterworth/3(Z_filt) -> [accBfFiltZ_g]  "accBfFiltZ"
  FilterButterworth/2(Y_filt) -> [accBfFiltY_g]  "accBfFiltY"
  FilterButterworth/1(X_filt) -> [accBfFiltX_g]  "accBfFiltX"
  [accBfY_g] -> FilterButterworth/2(Y)
  [StepTime] -> FilterButterworth/5(SampleTime)
  [accBfX_g] -> FilterButterworth/1(X)
  Sqrt/1 -> Goto63/1  "accXYFilt"
  Add2/1 -> Sqrt/1
  Math Function/1 -> Add2/1
  Math Function1/1 -> Add2/2
  [accBfFiltZ_g] -> TipOver/1(TO_curAccFiltZg)
  [SDO_fire] -> BikeCrashFusionProduct/9(CF_sdoFire)
  [eulerRoll_deg] -> Square/1
  Sqrt1/1 -> [tipOverAngle_deg]  "tipOverAngle_deg"
  1-D Lookup Table4/1 -> [GroundHitEnergyThreshold]  "GroundHitEnergyThresholdRoll"
  [GroundHitEnergyThreshold] -> HitDetection/21(HD_groundHitEnergyThreshold)
  Add5/1 -> Sqrt1/1
  Square/1 -> Add5/1
  [eulerPitch_deg] -> Square1/1
  Square1/1 -> Add5/2
  [SD_fire] -> SmartphoneDropOut_SDO/4(SDO_StandDetectionFire)
  [accBfZ_g] -> MATLAB Function/4(accBfZ_g)
  [accBfX_g] -> Add6/2, Switch5/3
  [accBfY_g] -> MATLAB Function/3(accBfY_g)
  [BMI_GYR_BF_X] -> MATLAB Function/5(gyrX_degs)
  [BMI_GYR_BF_Z] -> MATLAB Function/7(gyrZ_degs)
  MATLAB Function/1(pitch_deg) -> Data Type Conversion42/1  "pitchKalman_deg"
  [StepTime] -> MATLAB Function/1(timeStep_s)
  MATLAB Function/4(innovationRoll) -> Terminator1/1  "innovationRoll"
  Madgwick IMU MATLAB Function1/6(GyroBiasY) -> Terminator23/1  "gyroBiasMadgwickCrashY"
  Madgwick IMU MATLAB Function1/7(GyroBiasZ) -> Terminator24/1  "gyroBiasMadgwickCrashZ"
  Madgwick IMU MATLAB Function1/5(GyroBiasX) -> Terminator22/1  "gyroBiasMadgwickCrashX"
  [BMI_GYR_BF_Y] -> MATLAB Function/6(gyrY_degs)
  MATLAB Function/8(rollAcc) -> Math Function7/1  "rollAcc"
  MATLAB Function/9(gyrBiasX) -> [gyrXBias]  "gyrBiasXKalman"
  MATLAB Function/10(gyrBiasY) -> [gyrYBias]  "gyrBiasYKalman"
  From151/1 -> Madgwick IMU MATLAB Function1/9(SecondCalibrationDonePeriod)
  [reinitializeEulerEstimation] -> MATLAB Function/8(reinitializeFlag)
  [SD_fire] -> MATLAB Function/9(SD_fire)
  [HD_GroundHitFire] -> Unit Delay6/1
  [HD_CollisionFire] -> Unit Delay7/1
  Unit Delay6/1 -> MATLAB Function/10(HD_GroundHit)
  Unit Delay7/1 -> MATLAB Function/11(HD_CollisionHit)
  [CP_scenario] -> Data Type Conversion15/1
  [varSum] -> MATLAB Function/13(varSum)
  [accBfFiltY_g] -> MATLAB Function/15(accBfFiltY_g)
  [accBfFiltZ_g] -> MATLAB Function/16(accBfFiltZ_g)
  MATLAB Function/11(u1) -> Terminator4/1  "u1"
  [TO_fire] -> Unit Delay10/1
  Unit Delay10/1 -> MATLAB Function/12(TO_fire)
  [varSum] -> FilterButterworth/6("accVarSum ")
  [SecondCalibrationDelayed] -> MATLAB Function/17(secondCalibrationIsDone)
  SmartphoneDropOut_SDO/5(SDO_deltaRollExtrema_deg) -> Terminator13/1  "deltaRollExtrema"
  SmartphoneDropOut_SDO/6(SDO_deltaPitchExtrema_deg) -> Terminator14/1  "deltaPitchExtrema"
  SmartphoneDropOut_SDO/7(SDO_deltaRollPitch_deg) -> Terminator15/1  "deltaRollPitch"
  [varSum] -> SmartphoneDropOut_SDO/5(SDO_curAccVarXYZ)
  From107/1 -> Terminator37/1
  Math Function5/1 -> Add4/2
  [accImpulseX] -> Math Function4/1
  [accImpulseSTY] -> Math Function3/1
  Add3/1 -> Terminator43/1  "accEnergyStXYintern"
  Math Function3/1 -> Add3/2
  Add4/1 -> Terminator44/1  "accEnergyXYintern"
  Math Function2/1 -> Add3/1
  [accImpulseSTX] -> Math Function2/1
  Math Function4/1 -> Add4/1
  [accImpulseY] -> Math Function5/1
  [tipOverAngle_deg] -> 1-D Lookup Table4/1
  [tipOverAngle_deg] -> TipOver/5(TO_curTipOverAngle_deg)
  Divide3/1 -> Atan/1
  From193/1 -> Divide3/1
  From192/1 -> Switch7/3, Compare To Constant9/1
  Atan/1 -> Gain12/1
  Gain12/1 -> Abs4/1
  Abs4/1 -> Goto66/1  "accTipOverAngle"
  [AccTipOverAngle_deg] -> TipOver/7(TO_curAccTipOverAngle)
  SmartphoneDropOut_SDO/8(SDO_minAccVarSum) -> Terminator16/1  "SDO_minAccVarSum"
  Chart/2(RRO_rollIntegrationAngle) -> Terminator9/1  "rollIntegrationAngle"
  cobiSetup [0/1/2]/1 -> Data Type Conversion41/1  "COBI_hubSetup"
  Data Type Conversion41/1 -> [cobiHubSetup]
  MATLAB Function/2(roll_deg) -> Data Type Conversion14/1  "rollKalman_deg"
  MATLAB Function/7(pitchAcc) -> Math Function6/1  "pitchAcc"
  [validatedSpeed_kmh] -> SmartphoneDropOut_SDO/6(SDO_curSpeed_kmh)
  [CF_fire] -> Unit Delay/1
  Unit Delay/1 -> HitDetection/5(HD_crashFire)
  [cobiHubSetup] -> BikeCrashFusionProduct/10(CF_cobiHubSetup)
  Data Type Conversion14/1 -> [eulerRoll_deg]  "roll_deg"
  Data Type Conversion42/1 -> [eulerPitch_deg]  "pitch_deg"
  Constant7/1 -> RideDetection_RD/2(RD_curSpeedDerivative)
  [RD_fire] -> HitDetection/15(HD_curRideFire)
  From143/1 -> MATLAB Function1/9(probRRO)
  From146/1 -> MATLAB Function1/10(probSDO)
  MATLAB Function1/8(p_cc1x) -> Terminator33/1  "p_cc1x"
  MATLAB Function1/1(p_noCrash) -> Terminator32/1  "p_noCrash"
  MATLAB Function1/9(p_cc3x) -> Terminator34/1  "p_cc3x"
  From164/1 -> MATLAB Function1/14(cobiHubSetup)
  From145/1 -> MATLAB Function1/13(tipOverAngleFused_deg)
  MATLAB Function1/5(p_maxCrashClass) -> Goto52/1  "probCrashClass"
  MATLAB Function1/6(outputGeneralCrashClass) -> Goto4/1  "generalCrashClass"
  MATLAB Function1/7(p_generalCrashClass) -> Goto3/1  "p_generalCrashClass"
  MATLAB Function1/3(crashClass) -> Goto59/1  "mostPossibleClass"
  From142/1 -> MATLAB Function1/7(probNoseOver)
  From141/1 -> MATLAB Function1/6(probTipOver)
  From26/1 -> MATLAB Function1/8(probGroundHit)
  From25/1 -> MATLAB Function1/2(probRide2)
  From50/1 -> MATLAB Function1/4(probColl)
  MATLAB Function1/4(outputCrashClass) -> Goto50/1  "finalProbCrashClass"
  From163/1 -> MATLAB Function1/12(systemConfig)
  From162/1 -> MATLAB Function1/11(probHubConnection)
  From165/1 -> MATLAB Function1/15(secondCalibDoneDelayed)
  From49/1 -> MATLAB Function1/3(probSoftColl)
  From51/1 -> MATLAB Function1/5(probStrongColl)
  MATLAB Function1/2(p_crash) -> Goto51/1  "p_crash"
  From140/1 -> MATLAB Function1/1(probRide1)
  [CF_fire] -> CP_crashPlausiblizer/1(CP_crashFire)
  [SD_fire] -> CP_crashPlausiblizer/2(CP_standFire)
  CP_crashPlausiblizer/2(CP_fire) -> [CP_plausibleCrashFire]  "plausibleCrash"
  [tipOverAngle_deg] -> CP_crashPlausiblizer/5(CP_tipOverAngleFused_deg)
  [AccTipOverAngle_deg] -> CP_crashPlausiblizer/4(CP_tipOverAngleAcc_deg)
  [validatedSpeed_kmh] -> CP_crashPlausiblizer/3(CP_curSpeed_kmh)
  [CF_scenario] -> CP_crashPlausiblizer/6(CP_crashClass)
  CP_crashPlausiblizer/1(CP_crashAborted) -> [CP_abort]  "crashAborted"
  [CP_plausibleCrashFire] -> Data Type Conversion10/1
  [validatedCadence] -> CP_crashPlausiblizer/7(CP_curCadence)
  [StepTime] -> CP_crashPlausiblizer/8(CP_timeStep_s)
  [speedDerivative] -> CP_crashPlausiblizer/9(CP_curSpeedDerivative)
  [CF_scenario] -> CP_crashPlausiblizer/10(CP_curCrashClass)
  CP_crashPlausiblizer/3(CP_plausibleCrashClass) -> [CP_scenario]  "plausibleCrashClass"
  [accBfZ_g] -> MATLAB Function2/6(accZ)
  [accBfY_g] -> MATLAB Function2/5(accY)
  [accBfX_g] -> MATLAB Function2/4(accX)
  [BMI_GYR_BF_X] -> MATLAB Function2/1(gyrX)
  [BMI_GYR_BF_Z] -> MATLAB Function2/3(gyrZ)
  [BMI_GYR_BF_Y] -> MATLAB Function2/2(gyrY)
  MATLAB Function2/4(varGyrX) -> [gyrVarX]  "varGyrX"
  MATLAB Function2/5(varGyrY) -> [gyrVarY]  "varGyrY"
  MATLAB Function2/6(varGyrZ) -> [gyrVarZ]  "varGyrZ"
  [gyrVarX] -> Add7/1
  [gyrVarZ] -> Add7/3
  [gyrVarY] -> Add7/2
  Add7/1 -> [gyrVarSum]  "gyrVarSum"
  [gyrVarSum] -> 1-D Lookup Table1/1
  1-D Lookup Table1/1 -> [groundHitScaleFactor]  "variableGroundHitThresholdScale"
  [groundHitScaleFactor] -> HitDetection/22(HD_groundHitScaleFactor)
  From253/1 -> Math Function/1
  From254/1 -> Math Function1/1
  [eulerPitch_deg] -> Abs5/1
  Abs3/1 -> 1-D Lookup Table2/1
  Abs5/1 -> 1-D Lookup Table5/1
  Switch4/1 -> Relational Operator/2, Switch/3  "CollisionEnergyThresholdEuler"
  1-D Lookup Table5/1 -> Switch4/3  "CollisionEnergyThresholdPitch"
  1-D Lookup Table2/1 -> Relational Operator1/1, Switch4/1  "CollisionEnergyThresholdRoll"
  Relational Operator1/1 -> Switch4/2
  Data Type Conversion18/1 -> Terminator35/1  "DU_accBfXmg"
  accDuX [mg]/1 -> Data Type Conversion18/1  "DU_accBfXmg"
  accDuZ [mg]/1 -> Data Type Conversion34/1  "DU_accBfZmg"
  Data Type Conversion34/1 -> [duAccZ_mg]  "DU_accBfZmg"
  [cobiHubSetup] -> TipOver/8(TO_cobiHubSetup)
  [duAccZFilt_G] -> TipOver/9(TO_curDuAccZFiltG)
  Gain8/1 -> Transfer Fcn First Order1/1
  Transfer Fcn First Order1/1 -> Goto114/1  "duAccZFiltToG"
  From255/1 -> Gain8/1
  FilterButterworth/4(duZ_filt) -> [duAccZFilt_G]  "duAccZFilt"
  Gain9/1 -> FilterButterworth/4(duZ)  "duAccZ_g"
  [duAccZ_mg] -> Gain9/1
  [tipOverAngle_deg] -> HitDetection/23(HD_curTipOverAngle_deg)
  Add/1 -> Abs1/1
  [gyrYBias] -> Saturation/1
  Unit Delay3/1 -> Add/2
  Add8/1 -> Abs/1
  Unit Delay8/1 -> Add8/2
  [gyrXBias] -> Saturation1/1
  Saturation/1 -> Unit Delay3/1
  Saturation1/1 -> Unit Delay8/1
  BikeCrashFusionProduct/5(HD_CollisionHitFireIntern) -> Terminator41/1  "CollisionHitFireIntern"
  MATLAB Function/12(u2) -> Terminator5/1  "u2"
  Madgwick IMU MATLAB Function1/3(eulerYaw) -> Terminator20/1  "yaw_deg"
  [SecondCalibrationDone] -> risingEdgeTrigger_RET/1(RET_curValue)
  [calibrationDelayTime_s] -> risingEdgeTrigger_RET/2(RET_Latchtime)  "delayTime"
  risingEdgeTrigger_RET/2(RET_OutDelayed) -> [SecondCalibrationDelayed]  "secCalibDone Delayed"
  risingEdgeTrigger_RET/1(RET_output) -> [reinitializeEulerEstimation]  "reinitEulerEstimation"
  From73/1 -> 1-D Lookup Table/1
  CP_crashPlausiblizer/4(CP_intDistance_m) -> Terminator19/1  "CP_integratedDistance_m"
  HitDetection/8(HD_maxImpulseAmplitude) -> Terminator8/1  "HD_maxImpulseAmplitude"
  SmartphoneDropOut_SDO/9(SDO_bikeUpright) -> [SDO_bikeStillUpright]  "SDO_bikeUpright"
  [tipOverAngle_deg] -> SmartphoneDropOut_SDO/7(SDO_tipOverAngle_deg)
  Math Function7/1 -> Add9/2
  Math Function6/1 -> Add9/1
  Add9/1 -> Sqrt2/1
  Sqrt2/1 -> [AccTipOverAngle_deg]  "tipOverAcc_deg"
  [SDO_bikeStillUpright] -> BikeCrashFusionProduct/11(CF_bikeStillUpright)
  MATLAB Function6/10(p_cc1x) -> Terminator28/1  "p_cc1x"
  MATLAB Function6/1(p_noCrash) -> Terminator25/1  "p_noCrash"
  MATLAB Function6/8(probRide1FreezeDebug) -> Terminator26/1  "ride1Freeze"
  MATLAB Function6/12(p_cc3x) -> Terminator30/1  "p_cc3x"
  MATLAB Function6/9(probRide2FreezeDebug) -> Terminator27/1  "ride2Freeze"
  From277/1 -> MATLAB Function5/16(cobiHubSetup)
  From279/1 -> MATLAB Function5/17(curDuAccZFiltG)
  Divide/1 -> MATLAB Function5/3(accEnergyXY50ms)
  From276/1 -> Chart2/10(LP_bikeUpright)
  MATLAB Function5/3(probSoftCollision) -> Goto80/1  "p_softColl"
  From278/1 -> MATLAB Function5/15(systemConfig)
  From33/1 -> To Workspace27/1
  From177/1 -> MATLAB Function5/1(tipOverAngle_deg)
  Chart2/10(LP_probTipOverTimer) -> Goto68/1  "probTipOverTimer"
  From186/1 -> To Workspace4/1
  Chart2/8(LP_probNoseOverLatched) -> Goto93/1  "p_noseOverLatched"
  From238/1 -> MATLAB Function6/14(tipOverAngleAcc_deg)
  From251/1 -> MATLAB Function5/6(accVariance70msLatched)
  From250/1 -> Chart3/2(LF_curAccXYEnergy70ms)
  From185/1 -> Terminator36/1
  From234/1 -> MATLAB Function6/12(systemConfig)
  MATLAB Function6/13(p_cc20) -> Terminator31/1  "p_cc20"
  From262/1 -> To Workspace34/1
  From198/1 -> MATLAB Function5/12(pitch_deg)
  From225/1 -> MATLAB Function6/5(probStrongColl)
  From265/1 -> To Workspace35/1
  From243/1 -> To Workspace26/1
  From263/1 -> Chart3/3(LF_tipOverAngleFused)
  [RRO_fire] -> RRO_fire [0/1]/1, To Workspace33/1
  Chart3/3(LF_tipOverAngleFusedLatched) -> Goto35/1
  MATLAB Function6/6(outputGeneralCrashClass) -> Goto103/1  "generalCrashClass"
  MATLAB Function5/6(probRd2) -> Goto83/1  "p_rd2"
  From211/1 -> To Workspace28/1
  From69/1 -> To Workspace19/1
  From182/1 -> Divide/2
  From184/1 -> To Workspace29/1
  Chart2/6(LP_probRide1Latched) -> Goto90/1  "p_rd1Latched"
  From260/1 -> To Workspace32/1
  From259/1 -> To Workspace31/1
  From252/1 -> MATLAB Function5/5(accEnergyXY70msLatched)
  MATLAB Function5/12(speedDerivativeTransformedRd) -> Goto73/1
  From232/1 -> MATLAB Function6/10(probSDO)
  MATLAB Function5/17(accBfZTransformationTO2) -> Goto77/1
  From187/1 -> To Workspace1/1
  MATLAB Function5/5(probRd1) -> Goto82/1  "p_rd1"
  MATLAB Function5/8(probTipOver2) -> Goto85/1  "P_TO2"
  From112/1 -> Divide/1
  MATLAB Function6/4(outputCrashClass) -> Goto94/1  "finalProbCrashClass"
  Chart3/1(LF_accXYEnergy70msLatched) -> Goto111/1  "accXYEnergy70msLatched"
  From218/1 -> Chart2/7(LP_curProbRide2)
  From214/1 -> Chart2/4(LP_curProbStrongColl)
  Chart3/2(LF_accVariance70msLatched) -> Goto110/1  "accVariance70msLatched"
  From200/1 -> To Workspace8/1
  From188/1 -> To Workspace2/1
  From213/1 -> Chart2/1(LP_curProbColl)
  From196/1 -> MATLAB Function5/11(accTipOverAngle_deg)
  Chart2/2(LP_probGroundHitLatched) -> Goto89/1  "p_ghLatched"
  From201/1 -> To Workspace11/1
  From180/1 -> MATLAB Function5/7(secondCalibDone)
  From212/1 -> To Workspace20/1
  MATLAB Function6/7(p_generalCrashClass) -> Goto102/1  "p_generalCrashClass"
  From242/1 -> To Workspace25/1
  MATLAB Function5/11(speed2sTransformedRd) -> Goto72/1
  From205/1 -> To Workspace13/1
  From228/1 -> MATLAB Function6/7(probNoseOver)
  Chart2/9(LP_probRroLatched) -> Goto99/1
  From241/1 -> MATLAB Function6/16(cobiHubSetup)
  From204/1 -> To Workspace12/1
  MATLAB Function6/5(p_maxCrashClass) -> Goto97/1  "probCrashClass"
  From72/1 -> To Workspace30/1
  From236/1 -> To Workspace23/1
  From273/1 -> MATLAB Function6/15(probTipOverTimer)
  From224/1 -> MATLAB Function6/4(probColl)
  MATLAB Function6/2(p_crash) -> Goto96/1  "p_crash"
  MATLAB Function6/3(crashClass) -> Goto98/1  "mostPossibleClass"
  From233/1 -> MATLAB Function6/11(probHubConnection)
  From227/1 -> MATLAB Function6/6(probTipOver)
  From222/1 -> MATLAB Function6/8(probGroundHit)
  MATLAB Function5/15(pitchAngleTransformationTO2) -> Goto75/1
  From235/1 -> To Workspace22/1
  From244/1 -> MATLAB Function6/17(secondCalibDoneDelayed)
  From230/1 -> MATLAB Function6/13(tipOverAngleFused_deg)
  From231/1 -> To Workspace21/1
  MATLAB Function5/14(TipOverAngleAccTransformedTOl) -> Goto74/1
  From220/1 -> Chart2/6(LP_curProbNoseOver)
  MATLAB Function5/10(speedTransformedColl) -> Goto71/1
  From237/1 -> To Workspace24/1
  From223/1 -> MATLAB Function6/3(probSoftColl)
  From207/1 -> To Workspace15/1
  From202/1 -> To Workspace9/1
  From191/1 -> To Workspace5/1
  From203/1 -> To Workspace10/1
  Chart2/3(LP_probSoftCollLatched) -> Goto88/1  "p_softCollLatched"
  From194/1 -> To Workspace7/1
  From239/1 -> Chart2/9(LP_curProbRro)
  From195/1 -> To Workspace6/1
  From206/1 -> To Workspace14/1
  From219/1 -> Chart2/8(LP_curProbTipOver)
  From216/1 -> Chart2/3(LP_curProbGroundHit)
  From139/1 -> MATLAB Function5/2(speed_kmh)
  Chart2/1(LP_probRide2Latched) -> Goto91/1  "p_rd2Latched"
  From215/1 -> Chart2/2(LP_curProbSoftColl)
  MATLAB Function5/16(pitchRollRelationTransformationTO2) -> Goto76/1
  From209/1 -> To Workspace17/1
  From210/1 -> To Workspace18/1
  From208/1 -> To Workspace16/1
  MATLAB Function5/13(tipOverAngleFusedTransformedTOl) -> Goto67/1
  From199/1 -> MATLAB Function5/13(roll_deg)
  From179/1 -> MATLAB Function5/9(RollDeriv)
  Chart2/5(LP_probStrongCollLatched) -> Goto87/1  "p_strongCollLatched"
  MATLAB Function5/2(probStrongCollision) -> Goto79/1  "p_strongColl"
  MATLAB Function5/7(probTipOver12) -> Goto84/1  "p_TO12"
  From249/1 -> Chart3/1(LF_curAccVariance70ms)
  MATLAB Function5/1(probCollision) -> Goto78/1  "p_coll"
  From197/1 -> MATLAB Function5/14(accBfZfilt)
  From178/1 -> MATLAB Function5/8(accImpulseY)
  From226/1 -> MATLAB Function6/1(probRide1)
  MATLAB Function5/9(tipOverAngleTransformedColl) -> Goto70/1
  From217/1 -> Chart2/5(LP_curProbRide1)
  MATLAB Function6/11(p_cc11) -> Terminator29/1  "p_cc11"
  From229/1 -> MATLAB Function6/9(probRRO)
  MATLAB Function5/4(probGroundHit) -> Goto81/1  "p_groundHit"
  From221/1 -> MATLAB Function6/2(probRide2)
  From108/1 -> MATLAB Function5/4(accEnergyXY70ms)
  Chart2/4(LP_probCollLatched) -> Goto86/1  "p_CollLatched"
  Chart2/7(LP_probTipOverLatched) -> Goto92/1  "p_tipOverLatched"
  Data Type Conversion4/1 -> [StepTime]  "stepTime"
  Data Type Conversion6/1 -> [calibrationDelayTime_s]  "calibrationDelayTime"
  Constant3/1 -> Data Type Conversion6/1  "calibrationDelayTime_s"
  Data Type Conversion11/1 -> [longAccCompForEulerEstFlag]  "longAccCompForEulerEstFlag"
  Constant5/1 -> Environment Controller1/2  "longAccCompForEulerEstFlag"
  Constant6/1 -> Data Type Conversion12/1  "tipOverAngleThreshold_deg"
  Data Type Conversion12/1 -> [TipOverAngleThreshold_deg]  "TipOverAngleThreshold_deg"
  [TipOverAngleThreshold_deg] -> TipOver/10(TO_angleThresholdForTO1_deg)
  Data Type Conversion35/1 -> [TipOverMinAccZFiltNoseOver_g]  "TipOverMinAccZFiltNoseOver_g"
  Constant12/1 -> Data Type Conversion35/1  "tipOverMinAccZFiltNoseOver_g"
  [TipOverMinAccZFiltNoseOver_g] -> TipOver/12(TO_minAccZFiltNoseOver_g)
  Constant10/1 -> Data Type Conversion36/1  "tipOverAccZFiltTreshold_g"
  Data Type Conversion36/1 -> [TipOverAccZFiltTreshold_g]  "TipOverAccZFiltTreshold_g"
  [TipOverAccZFiltTreshold_g] -> TipOver/11(TO_accZFiltThreshold_g)
  Constant13/1 -> Data Type Conversion40/1  "tipOverRollPitchRelationNoseOver"
  Data Type Conversion40/1 -> [TipOverRollPitchRelationNoseOver]  "TipOverRollPitchRelationNoseOver"
  [TipOverRollPitchRelationNoseOver] -> TipOver/13(TO_rollPitchRelationNoseOver)
  Data Type Conversion22/1 -> [groundHitEnergyThresholdStanding_g2s2]  "groundHitEnergyThresholdStanding_g2s2"
  Constant14/1 -> Data Type Conversion22/1  "groundHitEnergyThresholdStanding_g2s2"
  Constant19/1 -> Data Type Conversion43/1  "groundHitTipOverAngleThreshold_deg"
  Data Type Conversion43/1 -> [groundHitTipOverAngleThreshold_deg]  "groundHitTipOverAngleThreshold_deg"
  [groundHitEnergyThresholdStanding_g2s2] -> HitDetection/24(HD_groundHitEnergyThresholdStanding)
  [groundHitTipOverAngleThreshold_deg] -> HitDetection/25(HD_groundHitAngleThreshold_deg)
  Constant20/1 -> Data Type Conversion44/1  "collisionVarianceThreshold_g2"
  Data Type Conversion44/1 -> [collisionVarianceThreshold_g2]  "collisionVarianceThreshold_g2"
  [collisionVarianceThreshold_g2] -> HitDetection/26(HD_collisionVarianceThreshold_g2)
  Data Type Conversion45/1 -> [strongHitSafetyFactor]  "strongHitSafetyFactor"
  Constant21/1 -> Data Type Conversion45/1  "strongHitSafetyFactor"
  [strongHitSafetyFactor] -> HitDetection/27(HD_strongHitSafetyfactor)
  Constant22/1 -> Data Type Conversion46/1  "scaleFactorVarianceStrongHit"
  Data Type Conversion46/1 -> [scaleFactorVarianceStrongHit]  "scaleFactorVarianceStrongHit"
  [scaleFactorVarianceStrongHit] -> HitDetection/28(HD_varScaleStrongHit)
  Data Type Conversion47/1 -> [minEnergyStrongHit_g2s2]  "minEnergyStrongHit_g2s2"
  Constant15/1 -> Data Type Conversion47/1  "minEnergyStrongHit_g2s2"
  [minEnergyStrongHit_g2s2] -> HitDetection/29(HD_minEnergyStrongHit_g2s2)
  Constant16/1 -> Data Type Conversion48/1  "collisionAngleThreshold_deg"
  Data Type Conversion48/1 -> [collisionAngleThreshold_deg]  "collisionAngleThreshold_deg"
  [collisionAngleThreshold_deg] -> HitDetection/30(HD_collisionAngleThreshold_deg)
  Data Type Conversion49/1 -> [noMotionAccVarianceThresholdSD_g2]  "noMotionAccVarianceThresholdSD_g2"
  Constant17/1 -> Data Type Conversion49/1  "noMotionAccVarianceThresholdSD_g2"
  [noMotionAccVarianceThresholdSD_g2] -> StandDetection_SD/3(SD_varianceThreshold_g2)
  Constant18/1 -> Data Type Conversion50/1  "ride1minSpeedSlow_kmh"
  Data Type Conversion50/1 -> [ride1minSpeedSlow_kmh]  "ride1minSpeedSlow_kmh"
  Data Type Conversion51/1 -> [ride2minSpeed_kmh]  "ride2minSpeed_kmh"
  Constant32/1 -> Data Type Conversion51/1  "ride2minSpeed_kmh"
  [ride1minSpeedSlow_kmh] -> RideDetection_RD/3(RD_minSpeedSlow)
  [ride2minSpeed_kmh] -> RideDetection_RD/4(RD_minSpeed)
  Data Type Conversion52/1 -> [rroMinGyrX_degs]  "rroMinGyrX_degs"
  Constant36/1 -> Data Type Conversion52/1  "rroMinGyrX_degs"
  [rroMinGyrX_degs] -> Chart/4(RRO_minGyroX_degs)
  Constant37/1 -> Data Type Conversion53/1  "rroUniContinuityThreshold_degs"
  Data Type Conversion53/1 -> [rroUniContinuityThreshold_degs]  "rroUniContinuityThreshold_degs"
  Constant38/1 -> Data Type Conversion54/1  "rroMaxSpeed_kmh"
  Data Type Conversion54/1 -> [rroMaxSpeed_kmh]  "rroMaxSpeed_kmh"
  Constant23/1 -> Data Type Conversion55/1  "rroMonotonyThreshold_degs"
  Data Type Conversion55/1 -> [rroMonotonyThreshold_degs]  "rroMonotonyThreshold_degs"
  Constant24/1 -> Data Type Conversion56/1  "rroRollIntegrationAngleThreshold_degs"
  Data Type Conversion56/1 -> [rroRollIntegrationAngleThreshold_degs]  "rroRollIntegrationAngleThreshold_degs"
  [rroUniContinuityThreshold_degs] -> Chart/5(RRO_uniContinuityThreshold_degs)
  [rroMaxSpeed_kmh] -> Chart/6(RRO_maxSpeed_kmh)
  [rroMonotonyThreshold_degs] -> Chart/7(RRO_monotonyThreshold_degs)
  [rroRollIntegrationAngleThreshold_degs] -> Chart/8(RRO_rollIntegrationAngleThreshold_degs)
  Data Type Conversion57/1 -> [sdoMaxTipOverAngle_deg]  "sdoMaxTipOverAngle_deg"
  Constant25/1 -> Data Type Conversion57/1  "sdoMaxTipOverAngle_deg"
  [sdoMaxTipOverAngle_deg] -> SmartphoneDropOut_SDO/8(SDO_maxTipOverAngle_deg)
  Data Type Conversion58/1 -> [sdoMinAccVar_g2]  "sdoMinAccVar_g2"
  Constant26/1 -> Data Type Conversion58/1  "sdoMinAccVar_g2"
  Data Type Conversion59/1 -> [sdoMinGyrXYNorm_degs]  "sdoMinGyrXYNorm_degs"
  Constant31/1 -> Data Type Conversion59/1  "sdoMinGyrXYNorm_degs"
  Constant33/1 -> Data Type Conversion60/1  "sdoMinOrientationChange_deg"
  Data Type Conversion60/1 -> [sdoMinOrientationChange_deg]  "sdoMinOrientationChange_deg"
  Constant34/1 -> Data Type Conversion61/1  "sdoScaleFactorOrientationChange"
  Data Type Conversion61/1 -> [sdoScaleFactorOrientationChange]  "sdoScaleFactorOrientationChange"
  Constant35/1 -> Data Type Conversion62/1  "sdoMaxAccVarFreeFall_g2"
  Data Type Conversion62/1 -> [sdoMaxAccVarFreeFall_g2]  "sdoMaxAccVarFreeFall_g2"
  Constant27/1 -> Data Type Conversion63/1  "sdoMinGyrXYNormFreeFall_degs"
  Data Type Conversion63/1 -> [sdoMinGyrXYNormFreeFall_degs]  "sdoMinGyrXYNormFreeFall_degs"
  [sdoMinGyrXYNormFreeFall_degs] -> SmartphoneDropOut_SDO/14(SDO_minGyrXYNormFreeFall_degs)
  [sdoMaxAccVarFreeFall_g2] -> SmartphoneDropOut_SDO/13(SDO_maxAccVarFreeFall_g2)
  [sdoScaleFactorOrientationChange] -> SmartphoneDropOut_SDO/12(SDO_scaleFactorOrientationChange)
  [sdoMinOrientationChange_deg] -> SmartphoneDropOut_SDO/11(SDO_minOrientationChange_deg)
  [sdoMinGyrXYNorm_degs] -> SmartphoneDropOut_SDO/10(SDO_minGyrXYNorm_degs)
  [sdoMinAccVar_g2] -> SmartphoneDropOut_SDO/9(SDO_minAccVar_g2)
  Constant43/1 -> Data Type Conversion67/1  "cpMinEstDistance_m"
  Constant44/1 -> Data Type Conversion68/1  "cpMinRiddenTime_s"
  Data Type Conversion67/1 -> [cpMinEstDistance_m]  "cpMinEstDistance_m"
  Data Type Conversion70/1 -> [cpSpeedCond2PositiveSpeedChangeTime_s]  "cpSpeedCond2PositiveSpeedChangeTime_s"
  Constant40/1 -> Data Type Conversion70/1  "cpSpeedCond2PositiveSpeedChangeTime_s"
  Constant29/1 -> Data Type Conversion65/1  "cpMinSpeedRiding_kmh"
  Data Type Conversion65/1 -> [cpMinSpeedRiding_kmh]  "cpMinSpeedRiding_kmh"
  Constant30/1 -> Data Type Conversion66/1  "cpNumCrankRevolutionThreshold"
  Data Type Conversion66/1 -> [cpNumCrankRevolutionThreshold]  "cpNumCrankRevolutionThreshold"
  Data Type Conversion64/1 -> [cpMaxAbortTime_s]  "cpMaxAbortTime_s"
  Constant39/1 -> Data Type Conversion69/1  "cpTimeOutSpeedCond2_s"
  Data Type Conversion69/1 -> [cpTimeOutSpeedCond2_s]  "cpTimeOutSpeedCond2_s"
  Constant28/1 -> Data Type Conversion64/1  "cpMaxAbortTime_s"
  Data Type Conversion68/1 -> [cpMinRiddenTime_s]  "cpMinRiddenTime_s"
  Constant41/1 -> Data Type Conversion71/1  "cpSpeedDerivativeThreshold_kmhs"
  Data Type Conversion71/1 -> [cpSpeedDerivativeThreshold_kmhs]  "cpSpeedDerivativeThreshold_kmhs"
  Data Type Conversion72/1 -> [cpMaxTipOverAngle_deg]  "cpMaxTipOverAngle_deg"
  Constant42/1 -> Data Type Conversion72/1  "cpMaxTipOverAngle_deg"
  [cpMaxAbortTime_s] -> CP_crashPlausiblizer/11(CP_maxAbortTime_s)
  [cpMaxTipOverAngle_deg] -> CP_crashPlausiblizer/19(CP_maxTipOverAngle_deg)
  [cpSpeedDerivativeThreshold_kmhs] -> CP_crashPlausiblizer/18(CP_speedDerivativeThreshold_kmhs)
  [cpSpeedCond2PositiveSpeedChangeTime_s] -> CP_crashPlausiblizer/17(CP_speedCond2PositiveSpeedChangeTime_s)
  [cpTimeOutSpeedCond2_s] -> CP_crashPlausiblizer/16(CP_timeOutSpeedCond2_s)
  [cpMinRiddenTime_s] -> CP_crashPlausiblizer/15(CP_minRiddenTime_s)
  [cpMinEstDistance_m] -> CP_crashPlausiblizer/14(CP_minEstDistance_m)
  [cpNumCrankRevolutionThreshold] -> CP_crashPlausiblizer/13(CP_numCrankRevolutionThreshold)
  [cpMinSpeedRiding_kmh] -> CP_crashPlausiblizer/12(CP_minSpeedRiding_kmh)
  MATLAB Function/3(innovationPitch) -> Terminator/1  "innovationPitch"
  MATLAB Function/5(pitchGyroPredict) -> Terminator2/1  "pitchGyroPredict"
  MATLAB Function/6(rollGyroPredict) -> Terminator3/1  "rollGyroPredict"
  [longAccCompForEulerEstFlag] -> Switch5/2
  Constant45/1 -> MATLAB Function5/10(speedDerivative)
  [SecondCalibrationDelayed] -> Data Type Conversion75/1
  Chart1/3(LAE_timer_s) -> Terminator39/1  "LAE_timer_s"
  [StepTime] -> Data Type Conversion76/1
  Data Type Conversion76/1 -> Chart1/6(LAE_timeStep_s)
  Data Type Conversion74/1 -> Chart1/4(LAE_curAccBfXFilt_g)
  Chart1/2(LAE_longAccTmp_g) -> Terminator38/1  "LAE_longAccTmp_g"
  Constant47/1 -> Chart1/3(LAE_minSpeedDelta_kmh)
  Data Type Conversion75/1 -> Chart1/5(LAE_curCalibState)
  [Du_Speed] -> Data Type Conversion73/1
  Chart1/1(LAE_longAcc_g) -> [longAccSpeedBased_g]  "LAE_longAcc_g"
  [accBfFiltX_g] -> Data Type Conversion74/1
  Data Type Conversion73/1 -> Chart1/2(LAE_curSpeed_kmh)
  Constant46/1 -> Chart1/1(LAE_minSpeed_kmh)
  Switch5/1 -> MATLAB Function/2(accBfX_g)
  Add6/1 -> Switch5/1
  [longAccSpeedBased_g] -> Add6/1
  Add10/1 -> Switch6/1
  [longAccSpeedBased_g] -> Add10/1
  [accBfFiltX_g] -> Add10/2, Switch6/3
  [longAccCompForEulerEstFlag] -> Switch6/2  "speedCompFlag"
  Switch6/1 -> MATLAB Function/14(accBfFiltX_g)
  Environment Controller1/1 -> Data Type Conversion11/1
  speedCompFlag [0/1]/1 -> Environment Controller1/1
  Switch7/1 -> Divide3/2
  Constant48/1 -> Switch7/1
  Compare To Constant9/1 -> Switch7/2
  [hubConnection] -> TipOver/14(TO_hubConnection)
  Constant49/1 -> Relational Operator1/2
  [hubConnection] -> Compare To Constant6/1
  Constant11/1 -> Switch3/1
  Compare To Constant7/1 -> Logical Operator2/1
  Compare To Constant6/1 -> Logical Operator2/2
  [SystemConfig] -> Compare To Constant7/1
  Compare To Constant8/1 -> Logical Operator2/3
  [cobiHubSetup] -> Compare To Constant8/1
  [Du_Speed] -> Switch3/3
  Logical Operator2/1 -> Switch2/2, Switch3/2
  Constant9/1 -> Switch2/1
  [Du_Cadence] -> Switch2/3
  Switch2/1 -> [validatedCadence]
  [validatedSpeed_kmh] -> RideDetection_RD/1(RD_curSpeed)
  Compare To Constant3/1 -> Logical Operator/2
  Unit Delay9/1 -> Switch1/1, Compare To Constant4/1
  Switch3/1 -> Switch1/3, Unit Delay9/1, Compare To Constant3/1, Goto154/1
  Logical Operator/1 -> Switch1/2
  Compare To Constant4/1 -> Logical Operator/1
  Switch1/1 -> [validatedSpeed_kmh]  "validatedSpeed_kmh"
  [ride1minSpeedSlow_kmh] -> SmartphoneDropOut_SDO/15(SDO_ride1minSpeed_kmh)
  [SystemConfig] -> RideDetection_RD/6(RD_systemConfig)
  [hubConnection] -> RideDetection_RD/5(RD_hubConnection)
  [cobiHubSetup] -> RideDetection_RD/7(RD_cobiHubSetup)
  Data Type Conversion77/1 -> [cpMinEstDistanceGnssBased_m]  "cpMinEstDistanceGnssBased_m"
  Constant8/1 -> Data Type Conversion77/1  "cpMinEstDistanceGnssBased_m"
  [cpMinEstDistanceGnssBased_m] -> CP_crashPlausiblizer/21(CP_minEstDistanceGnssBased_m)
  [cobiHubSetup] -> CP_crashPlausiblizer/20(CP_hubSetup)
  CP_crashPlausiblizer/5(CP_intDistanceGnssBased_m) -> Terminator42/1  "CP_integratedDistanceGnssBased_m"
